simulink model "asbQuadcopters_SiFi"  (Simulink 9.1)
settings: Solver=VariableStepAuto  StartTime=0.0  StopTime=TFinal  RelTol=1e-3
values from neighbouring files (symbols this model uses):
  Controller =     [data_set.mat]
  Estimator =     [data_set.mat]
  g = 9.81    [data_set.mat]
  init =     [data_set.mat]
  rho = 1.184    [data_set.mat]
  sensorCalibrationData = [0.09 -0.06 -9.473 -0.0095 -0.0075 0.0015 101270.95 0.2]    [data_set.mat]
  Sensors =     [data_set.mat]
  States =     [data_set.mat]
  takeOffDuration = 1    [data_set.mat]
  Ts = 0.005    [data_set.mat]
  Vehicle =     [data_set.mat]
undefined symbols (not defined in the file or in its folder): DiscIntNeverNeededParam, Discrete, Earth, ft, m, s, sigbuilder_block, Time, WGS84
libraries: F_Line_block x565, simulink x39, aerolibconvert2 x4, sharedutil x3, ctrlSharedLib x3, sharedtransform x3, shared6dof x1, aerolibasang x1, aerolibtransform2 x1, aerolibnav x1, aerolibanimutils x1
(part 3 of 4)

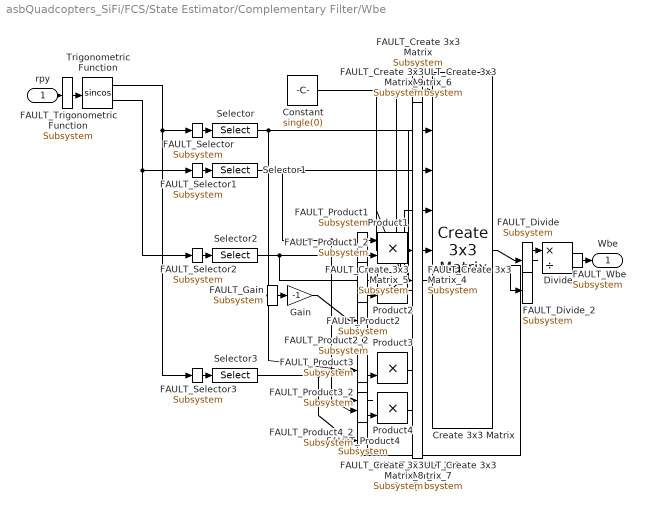
== system asbQuadcopters_SiFi/FCS/State Estimator/Complementary Filter/Wbe ==
  rpy : Inport  OutDataTypeStr=single
  Constant : Constant  Value=single(0)
  Create 3x3 Matrix : sharedutil/Create 3x3 Matrix  aMode=aMode
  FAULT_Create 3x3 Matrix : F_Line_block/Subsystem
  FAULT_Create 3x3 Matrix_{2..9} (8 alike) : F_Line_block/Subsystem
  Divide : Product  Inputs=*/
  FAULT_Divide : F_Line_block/Subsystem
  FAULT_Divide_2 : F_Line_block/Subsystem
  Gain : Gain  Gain=-1
  FAULT_Gain : F_Line_block/Subsystem
  Product{1..4} (4 alike) : Product
  FAULT_Product{1..4} (4 alike) : F_Line_block/Subsystem
  FAULT_Product1_2 : F_Line_block/Subsystem
  FAULT_Product2_2 : F_Line_block/Subsystem
  FAULT_Product3_2 : F_Line_block/Subsystem
  FAULT_Product4_2 : F_Line_block/Subsystem
  Selector : Selector  InputPortWidth=3  IndexOptions=Index vector (dialog)  Indices=[1]  OutputSizes=1
  FAULT_Selector{,1..3} (4 alike) : F_Line_block/Subsystem
  Selector1 : Selector  InputPortWidth=3  IndexOptions=Index vector (dialog)  Indices=[1]  OutputSizes=1
  Selector2 : Selector  InputPortWidth=3  IndexOptions=Index vector (dialog)  Indices=[2]  OutputSizes=1
  Selector3 : Selector  InputPortWidth=3  IndexOptions=Index vector (dialog)  Indices=[2]  OutputSizes=1
  Trigonometric Function : Trigonometry  Operator=sincos
  FAULT_Trigonometric Function : F_Line_block/Subsystem
  Wbe : Outport
  FAULT_Wbe : F_Line_block/Subsystem
  wires:
  Create 3x3 Matrix/1 -> FAULT_Divide/1
  FAULT_Divide/1 -> Divide/1
  Product3/1 -> ?
  FAULT_Create 3x3 Matrix/1 -> Create 3x3 Matrix/1
  Trigonometric Function/2 -> FAULT_Selector1/1, FAULT_Selector2/1
  FAULT_Selector1/1 -> Selector1/1
  FAULT_Selector2/1 -> Selector2/1
  Selector3/1 -> FAULT_Product4_2/1, FAULT_Product3_2/1
  FAULT_Product4_2/1 -> Product4/2
  FAULT_Product3_2/1 -> Product3/2
  Selector1/1 -> FAULT_Product4/1, Product1/1, Create 3x3 Matrix/3
  Trigonometric Function/1 -> FAULT_Selector3/1, FAULT_Selector/1
  FAULT_Selector3/1 -> Selector3/1
  FAULT_Selector/1 -> Selector/1
  Product1/1 -> FAULT_Create 3x3 Matrix_5/1
  FAULT_Create 3x3 Matrix_5/1 -> Create 3x3 Matrix/5
  Product2/1 -> ?
  FAULT_Create 3x3 Matrix_5/1 -> Create 3x3 Matrix/5
  Selector2/1 -> FAULT_Divide_2/1, Product2/1, Product1/2
  Gain/1 -> FAULT_Product2_2/1
  FAULT_Product2_2/1 -> Product2/2
  Product4/1 -> ?
  FAULT_Create 3x3 Matrix_2/1 -> Create 3x3 Matrix/2
  Constant/1 -> FAULT_Create 3x3 Matrix_4/1, FAULT_Create 3x3 Matrix/1
  FAULT_Create 3x3 Matrix_4/1 -> Create 3x3 Matrix/4
  FAULT_Create 3x3 Matrix/1 -> Create 3x3 Matrix/1
  Divide/1 -> FAULT_Wbe/1
  FAULT_Wbe/1 -> Wbe/1
  rpy/1 -> FAULT_Trigonometric Function/1
  FAULT_Trigonometric Function/1 -> Trigonometric Function/1
  Selector/1 -> FAULT_Product3/1, Gain/1, Create 3x3 Matrix/2

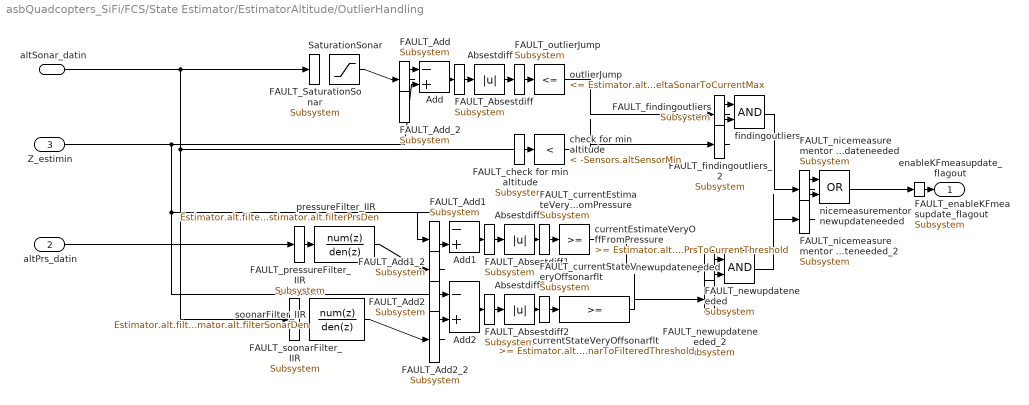
== system asbQuadcopters_SiFi/FCS/State Estimator/EstimatorAltitude/OutlierHandling ==
  altSonar_datin : Inport
  altPrs_datin : Inport  Port=2
  Z_estimin : Inport  Port=3
  Absestdiff : Abs
  FAULT_Absestdiff : F_Line_block/Subsystem
  Absestdiff1 : Abs
  FAULT_Absestdiff1 : F_Line_block/Subsystem
  Absestdiff2 : Abs
  FAULT_Absestdiff2 : F_Line_block/Subsystem
  Add : Sum  Inputs=-+
  FAULT_Add : F_Line_block/Subsystem
  FAULT_Add_2 : F_Line_block/Subsystem
  Add1 : Sum  Inputs=-+
  FAULT_Add1 : F_Line_block/Subsystem
  FAULT_Add1_2 : F_Line_block/Subsystem
  Add2 : Sum  Inputs=-+
  FAULT_Add2 : F_Line_block/Subsystem
  FAULT_Add2_2 : F_Line_block/Subsystem
  SaturationSonar : Saturate  UpperLimit=-Sensors.altSensorMin  LowerLimit=-inf
  FAULT_SaturationSonar : F_Line_block/Subsystem
  check for min altitude : simulink/Logic and Bit Operations/Compare To Constant  relop=<  const=-Sensors.altSensorMin  OutDataTypeStr=boolean
  FAULT_check for min altitude : F_Line_block/Subsystem
  currentEstimateVeryOffFromPressure : simulink/Logic and Bit Operations/Compare To Constant  relop=>=  const=Estimator.alt.deltaPrsToCurrentThreshold  OutDataTypeStr=boolean
  FAULT_currentEstimateVeryOffFromPressure : F_Line_block/Subsystem
  currentStateVeryOffsonarflt : simulink/Logic and Bit Operations/Compare To Constant  relop=>=  const=Estimator.alt.deltaSonarToFilteredThreshold  OutDataTypeStr=boolean
  FAULT_currentStateVeryOffsonarflt : F_Line_block/Subsystem
  findingoutliers : Logic  AllPortsSameDT=off  OutDataTypeStr=boolean
  FAULT_findingoutliers : F_Line_block/Subsystem
  FAULT_findingoutliers_2 : F_Line_block/Subsystem
  newupdateneeded : Logic  AllPortsSameDT=off  OutDataTypeStr=boolean
  FAULT_newupdateneeded : F_Line_block/Subsystem
  FAULT_newupdateneeded_2 : F_Line_block/Subsystem
  nicemeasurementor newupdateneeded : Logic  Operator=OR  AllPortsSameDT=off  OutDataTypeStr=boolean
  FAULT_nicemeasurementor newupdateneeded : F_Line_block/Subsystem
  FAULT_nicemeasurementor newupdateneeded_2 : F_Line_block/Subsystem
  outlierJump : simulink/Logic and Bit Operations/Compare To Constant  relop=<=  const=Estimator.alt.deltaSonarToCurrentMax  OutDataTypeStr=boolean
  FAULT_outlierJump : F_Line_block/Subsystem
  pressureFilter_IIR : DiscreteFilter  Numerator=Estimator.alt.filterPrsNum  Denominator=Estimator.alt.filterPrsDen
  FAULT_pressureFilter_IIR : F_Line_block/Subsystem
  soonarFilter_IIR : DiscreteFilter  Numerator=Estimator.alt.filterSonarNum  Denominator=Estimator.alt.filterSonarDen
  FAULT_soonarFilter_IIR : F_Line_block/Subsystem
  enableKFmeasupdate_flagout : Outport
  FAULT_enableKFmeasupdate_flagout : F_Line_block/Subsystem
  wires:
  Add1/1 -> FAULT_Absestdiff1/1
  FAULT_Absestdiff1/1 -> Absestdiff1/1
  nicemeasurementor newupdateneeded/1 -> FAULT_enableKFmeasupdate_flagout/1
  FAULT_enableKFmeasupdate_flagout/1 -> enableKFmeasupdate_flagout/1
  findingoutliers/1 -> FAULT_nicemeasurementor newupdateneeded/1
  FAULT_nicemeasurementor newupdateneeded/1 -> nicemeasurementor newupdateneeded/1
  check for min altitude/1 -> FAULT_findingoutliers_2/1
  FAULT_findingoutliers_2/1 -> findingoutliers/2
  outlierJump/1 -> FAULT_findingoutliers/1
  FAULT_findingoutliers/1 -> findingoutliers/1
  SaturationSonar/1 -> FAULT_Add/1
  FAULT_Add/1 -> Add/1
  Absestdiff/1 -> FAULT_outlierJump/1
  FAULT_outlierJump/1 -> outlierJump/1
  Add/1 -> FAULT_Absestdiff/1
  FAULT_Absestdiff/1 -> Absestdiff/1
  newupdateneeded/1 -> FAULT_nicemeasurementor newupdateneeded_2/1
  FAULT_nicemeasurementor newupdateneeded_2/1 -> nicemeasurementor newupdateneeded/2
  Absestdiff2/1 -> FAULT_currentStateVeryOffsonarflt/1
  FAULT_currentStateVeryOffsonarflt/1 -> currentStateVeryOffsonarflt/1
  altSonar_datin/1 -> FAULT_SaturationSonar/1, FAULT_soonarFilter_IIR/1, check for min altitude/1
  currentEstimateVeryOffFromPressure/1 -> FAULT_newupdateneeded/1
  FAULT_newupdateneeded/1 -> newupdateneeded/1
  Z_estimin/1 -> FAULT_Add1/1, Add2/1, Add/2
  Add2/1 -> FAULT_Absestdiff2/1
  FAULT_Absestdiff2/1 -> Absestdiff2/1
  currentStateVeryOffsonarflt/1 -> FAULT_newupdateneeded_2/1
  FAULT_newupdateneeded_2/1 -> newupdateneeded/2
  pressureFilter_IIR/1 -> FAULT_Add1_2/1
  FAULT_Add1_2/1 -> Add1/2
  altPrs_datin/1 -> FAULT_pressureFilter_IIR/1
  FAULT_pressureFilter_IIR/1 -> pressureFilter_IIR/1
  soonarFilter_IIR/1 -> FAULT_Add2_2/1
  FAULT_Add2_2/1 -> Add2/2
  Absestdiff1/1 -> FAULT_currentEstimateVeryOffFromPressure/1
  FAULT_currentEstimateVeryOffFromPressure/1 -> currentEstimateVeryOffFromPressure/1

== system asbQuadcopters_SiFi/FCS/State Estimator/EstimatorXYPosition/EstimatorVelocity ==
  opticalFlow_datin : Inport
  Z_estimin : Inport  Port=2  SampleTime=Ts
  sensorIMU_datin : Inport  Port=3
  orient_estimin : Inport  Port=4
  AccelerationHandling : Subsystem
  DataHandling : Subsystem
  Delay : Delay  DelayLength=1  InitialCondition=0
  FAULT_Delay : F_Line_block/Subsystem
  KalmanFilter_dxdy : ctrlSharedLib/Kalman Filter  TimeDomain=Discrete-Time  UseCurrentEstimator=on  ModelSource=Individual A, B, C, D matrices  ModelSourceVariable=ss(0.95,1,1,0,1)  A=eye(2)  B=Ts*eye(2)  C=eye(2)  D=0  NumberOfStates=1  NumberOfInputs=1  NumberOfOutputs=1  InitialEstimateSource=Dialog  X0=0  P0=10  UseK=off  UseGH=on  NumberOfProcessNoiseInputs=1  G=Estimator.pos.kfVelo.G  TimeInvariantG=on  H=Estimator.pos.kfVelo.H  TimeInvariantH=on  Q=Estimator.pos.kfVelo.Q  TimeInvariantQ=on  R=Estimator.pos.kfVelo.R  TimeInvariantR=on  N=Estimator.pos.kfVelo.N  TimeInvariantN=on  AddInputPort=on  AddEnablePort=on  OutputEstimatedY=off  OutputP=off  Ts=-1
      settings: SourceProductBaseCode=CT
  FAULT_KalmanFilter_dxdy : F_Line_block/Subsystem
  FAULT_KalmanFilter_dxdy_2 : F_Line_block/Subsystem
  FAULT_KalmanFilter_dxdy_3 : F_Line_block/Subsystem
  Select dxy : Selector  InputPortWidth=3  IndexOptions=Index vector (dialog)  Indices=[1 2]  OutputSizes=1
  FAULT_Select dxy : F_Line_block/Subsystem
  opticalFlowToVelocity_gain : Gain  Gain=Estimator.pos.opticalFlowToVelocityGain
  FAULT_opticalFlowToVelocity_gain : F_Line_block/Subsystem
  dxy_estimout : Outport
  FAULT_dxy_estimout : F_Line_block/Subsystem
  wires:
  Delay/1 -> DataHandling/5(dxyOF_datin)
  Z_estimin/1 -> DataHandling/1(Z_estimin), AccelerationHandling/4(Z_estimin)
  KalmanFilter_dxdy/1 -> FAULT_dxy_estimout/1, FAULT_Delay/1
  ?FAULT_Demux1/1 -> ?Demux1/1
  ?FAULT_IIRgyroz/1 -> ?IIRgyroz/1
  FAULT_dxy_estimout/1 -> dxy_estimout/1
  FAULT_Delay/1 -> Delay/1
  opticalFlowToVelocity_gain/1 -> FAULT_Select dxy/1
  FAULT_Select dxy/1 -> Select dxy/1
  opticalFlow_datin/1 -> FAULT_opticalFlowToVelocity_gain/1
  FAULT_opticalFlowToVelocity_gain/1 -> opticalFlowToVelocity_gain/1
  sensorIMU_datin/1 -> AccelerationHandling/2(sensorIMU_datin), DataHandling/3(sensorIMU_datin)
  orient_estimin/1 -> AccelerationHandling/3(orient_estimin), DataHandling/2(orient_estimin)
  Select dxy/1 -> FAULT_KalmanFilter_dxdy_2/1, AccelerationHandling/1(dxy_estimin), DataHandling/4(dxy_estimin)
  AccelerationHandling/1(acceleration_world) -> FAULT_KalmanFilter_dxdy/1
  FAULT_KalmanFilter_dxdy/1 -> KalmanFilter_dxdy/1
  DataHandling/1(enable_flag) -> FAULT_KalmanFilter_dxdy_3/1
  FAULT_KalmanFilter_dxdy_3/1 -> KalmanFilter_dxdy/3

== system asbQuadcopters_SiFi/FCS/State Estimator/EstimatorXYPosition/EstimatorXYPosition ==
  note: Switching from orientationControl to Position
      | control reset the current world position estimate
      | (happens when using no markers)
  dxy_estimin : Inport
  orient_estimin : Inport  Port=2  SampleTime=Ts
  controlModePosVSOrient_flagin : Inport  Port=3
  dz_estimin : Inport  Port=4
  posVIS_datin : Inport  Port=5
  usePosVIS_flagin : Inport  Port=6
  Delay : Delay  DelayLength=1  InitialCondition=0
  FAULT_Delay : F_Line_block/Subsystem
  KalmanFilter_posxy : ctrlSharedLib/Kalman Filter  TimeDomain=Discrete-Time  UseCurrentEstimator=on  ModelSource=Individual A, B, C, D matrices  ModelSourceVariable=ss(0.95,1,1,0,1)  A=eye(2)  B=Ts*eye(2)  C=eye(2)  D=0  NumberOfStates=1  NumberOfInputs=1  NumberOfOutputs=1  InitialEstimateSource=Dialog  X0=[.1 0]  P0=10  UseK=off  UseGH=on  NumberOfProcessNoiseInputs=1  G=Estimator.pos.kfPos.G  TimeInvariantG=on  H=Estimator.pos.kfPos.H  TimeInvariantH=on  Q=Estimator.pos.kfPos.Q  TimeInvariantQ=on  R=Estimator.pos.kfPos.R  TimeInvariantR=on  N=Estimator.pos.kfPos.N  TimeInvariantN=on  AddInputPort=on  AddEnablePort=on  OutputEstimatedY=off  OutputP=off  Ts=-1
      settings: SourceProductBaseCode=CT
  FAULT_KalmanFilter_posxy : F_Line_block/Subsystem
  FAULT_KalmanFilter_posxy_2 : F_Line_block/Subsystem
  FAULT_KalmanFilter_posxy_3 : F_Line_block/Subsystem
  Math Function : Math  Operator=transpose  SaturateOnIntegerOverflow=on
  FAULT_Math Function : F_Line_block/Subsystem
  Mux2 : Mux  Inputs=2
  FAULT_Mux2 : F_Line_block/Subsystem
  FAULT_Mux2_2 : F_Line_block/Subsystem
  OutlierHandling : Subsystem
  Product : Product  Multiplication=Matrix(*)
  FAULT_Product : F_Line_block/Subsystem
  FAULT_Product_2 : F_Line_block/Subsystem
  Rotation Angles to Direction Cosine Matrix : sharedtransform/Rotation Angles to Direction Cosine Matrix  rotationOrder=ZYX  aMode=aMode
      settings: SourceProductBaseCode=AE
  FAULT_Rotation Angles to Direction Cosine Matrix : F_Line_block/Subsystem
  SelectXY : Selector  InputPortWidth=4  IndexOptions=Index vector (dialog)  Indices=[1 2]  OutputSizes=1
  FAULT_SelectXY : F_Line_block/Subsystem
  SelectdXY : Selector  InputPortWidth=3  IndexOptions=Index vector (dialog)  Indices=[1 2]  OutputSizes=1
  FAULT_SelectdXY : F_Line_block/Subsystem
  SimplyIntegrateVelocity : DiscreteIntegrator  ExternalReset=rising  SampleTime=Ts  ICPrevOutput=DiscIntNeverNeededParam  ICPrevScaledInput=DiscIntNeverNeededParam
  FAULT_SimplyIntegrateVelocity : F_Line_block/Subsystem
  FAULT_SimplyIntegrateVelocity_2 : F_Line_block/Subsystem
  UseIPPosSwitch : Switch  Criteria=u2 > Threshold
  XY_estimout : Outport
  FAULT_XY_estimout : F_Line_block/Subsystem
  wires:
  Delay/1 -> OutlierHandling/3(pos_estim)
  usePosVIS_flagin/1 -> UseIPPosSwitch/2
  UseIPPosSwitch/1 -> FAULT_XY_estimout/1
  FAULT_XY_estimout/1 -> XY_estimout/1
  controlModePosVSOrient_flagin/1 -> FAULT_SimplyIntegrateVelocity_2/1
  FAULT_SimplyIntegrateVelocity_2/1 -> SimplyIntegrateVelocity/2
  KalmanFilter_posxy/1 -> FAULT_Delay/1, UseIPPosSwitch/1
  FAULT_Delay/1 -> Delay/1
  FAULT_SelectXY/1 -> SelectXY/1
  posVIS_datin/1 -> OutlierHandling/2(posVIS_datin), FAULT_SelectXY/1
  FAULT_Delay/1 -> Delay/1
  FAULT_SelectXY/1 -> SelectXY/1
  Product/1 -> FAULT_SelectdXY/1
  FAULT_SelectdXY/1 -> SelectdXY/1
  Mux2/1 -> FAULT_Product_2/1
  FAULT_Product_2/1 -> Product/2
  dz_estimin/1 -> FAULT_Mux2_2/1
  FAULT_Mux2_2/1 -> Mux2/2
  SimplyIntegrateVelocity/1 -> UseIPPosSwitch/3
  dxy_estimin/1 -> FAULT_Mux2/1
  FAULT_Mux2/1 -> Mux2/1
  orient_estimin/1 -> FAULT_Rotation Angles to Direction Cosine Matrix/1, OutlierHandling/1(orient_estimin)
  FAULT_Rotation Angles to Direction Cosine Matrix/1 -> Rotation Angles to Direction Cosine Matrix/1
  FAULT_SelectXY/1 -> SelectXY/1
  Rotation Angles to Direction Cosine Matrix/1 -> FAULT_Math Function/1
  FAULT_Math Function/1 -> Math Function/1
  SelectXY/1 -> FAULT_KalmanFilter_posxy_2/1
  FAULT_KalmanFilter_posxy_2/1 -> KalmanFilter_posxy/2
  OutlierHandling/1(enable_flag) -> FAULT_KalmanFilter_posxy_3/1
  FAULT_KalmanFilter_posxy_3/1 -> KalmanFilter_posxy/3
  SelectdXY/1 -> FAULT_SimplyIntegrateVelocity/1, FAULT_KalmanFilter_posxy/1
  FAULT_SimplyIntegrateVelocity/1 -> SimplyIntegrateVelocity/1
  FAULT_KalmanFilter_posxy/1 -> KalmanFilter_posxy/1
  Math Function/1 -> FAULT_Product/1
  FAULT_Product/1 -> Product/1

== system asbQuadcopters_SiFi/Sensor/Sensor System/IMU_Pressure/HAL_acquisition_creator ==
  sensors : Inport
  Bus Creator4 : BusCreator  Inputs=21  OutDataTypeStr=Bus: HAL_acquisition_t  NonVirtualBus=on
      settings: InheritFromInputs=off
  Demux3 : Demux  Outputs=8
  HAL_acc_SI_creator : Subsystem
  HAL_fifo_fsync : Constant  Value=zeros(5,1)  OutDataTypeStr=uint8
  HAL_fifo_gyro_SI_t_creator : Subsystem
  HAL_fifo_gyro_SI_t_creator1 : Subsystem
  HAL_fifo_gyro_SI_t_creator2 : Subsystem
  HAL_fifo_gyro_SI_t_creator3 : Subsystem
  HAL_gyro_SI_creator : Subsystem
  HAL_magn_mG_t_creator1 : Subsystem
  HAL_pressure_SI_creator : Subsystem
  HAL_ultrasound_SI_creator : Subsystem
  HAL_vbat_SI_creator : Subsystem
  number_HAL_read_call : Constant  Value=0  OutDataTypeStr=int32
  number_HAL_read_call1 : Constant  Value=0  OutDataTypeStr=uint32
  number_HAL_read_call2 : Constant  Value=0  OutDataTypeStr=uint16
  number_HAL_read_call3 : Constant  Value=0  OutDataTypeStr=uint8
  number_HAL_read_call4 : Constant  Value=0  OutDataTypeStr=uint8
  number_HAL_read_call5 : Constant  Value=0  OutDataTypeStr=uint16
  number_HAL_read_call6 : Constant  Value=0  OutDataTypeStr=uint32
  number_HAL_read_call7 : Constant  Value=0  OutDataTypeStr=single
  number_HAL_read_call8 : Constant  Value=0  OutDataTypeStr=int32
  padding : Constant  Value=zeros(1,196)  OutDataTypeStr=uint8
  HAL_acquisition_t : Outport  OutDataTypeStr=Bus: HAL_acquisition_t
  wires:
  Demux3/4 -> HAL_gyro_SI_creator/1(x)  "x"
  HAL_gyro_SI_creator/1(HAL_gyro_SI) -> Bus Creator4/7  "HAL_gyro_SI"
  Demux3/7 -> HAL_ultrasound_SI_creator/1(altitude)  "altitude"
  HAL_fifo_gyro_SI_t_creator2/1(HAL_fifo_gyro_SI_TempCorr) -> Bus Creator4/12  "HAL_fifo_gyro_SI"
  HAL_magn_mG_t_creator1/1(HAL_magn_mG) -> Bus Creator4/17  "HAL_magn_mG"
  HAL_vbat_SI_creator/1(HAL_vbat_SI) -> Bus Creator4/21  "HAL_vbat_SI"
  sensors/1 -> Demux3/1
  number_HAL_read_call4/1 -> Bus Creator4/5  "count_user"
  Demux3/5 -> HAL_gyro_SI_creator/2(y)  "y"
  number_HAL_read_call8/1 -> Bus Creator4/16  "HAL_fifo_size"
  HAL_fifo_gyro_SI_t_creator1/1(HAL_fifo_acce_SI_TempCorr) -> Bus Creator4/11  "HAL_fifo_acce_SI_TempCorr"
  Demux3/6 -> HAL_gyro_SI_creator/3(z)  "z"
  Demux3/8 -> HAL_pressure_SI_creator/1(pressure)  "pressure"
  number_HAL_read_call/1 -> Bus Creator4/1  "number_HAL_read_call"
  number_HAL_read_call6/1 -> Bus Creator4/9  "fifo_timestamp"
  number_HAL_read_call3/1 -> Bus Creator4/4  "used"
  number_HAL_read_call5/1 -> Bus Creator4/8  "HAL_fifo_count"
  Demux3/2 -> HAL_acc_SI_creator/2(y)  "y"
  number_HAL_read_call2/1 -> Bus Creator4/3  "status"
  Demux3/1 -> HAL_acc_SI_creator/1(x)  "x"
  padding/1 -> Bus Creator4/20  "padding"
  HAL_fifo_fsync/1 -> Bus Creator4/15  "HAL_fifo_fsync"
  number_HAL_read_call7/1 -> Bus Creator4/14  "HAL_ref_IMU_temp"
  number_HAL_read_call1/1 -> Bus Creator4/2  "timestamp"
  HAL_fifo_gyro_SI_t_creator3/1(HAL_fifo_acce_SI_TempCorr) -> Bus Creator4/13  "HAL_fifo_acce_SI"
  HAL_acc_SI_creator/1(HAL_acc_SI) -> Bus Creator4/6  "HAL_acc_SI"
  HAL_fifo_gyro_SI_t_creator/1(HAL_fifo_gyro_SI_TempCorr) -> Bus Creator4/10  "HAL_fifo_gyro_SI_TempCorr"
  Demux3/3 -> HAL_acc_SI_creator/3(z)  "z"
  HAL_pressure_SI_creator/1(HAL_pressure_SI) -> Bus Creator4/18  "HAL_pressure_SI"
  Bus Creator4/1 -> HAL_acquisition_t/1  "HAL_acquisition_t"
  HAL_ultrasound_SI_creator/1(HAL_ultrasound_SI) -> Bus Creator4/19  "HAL_ultrasound_SI"

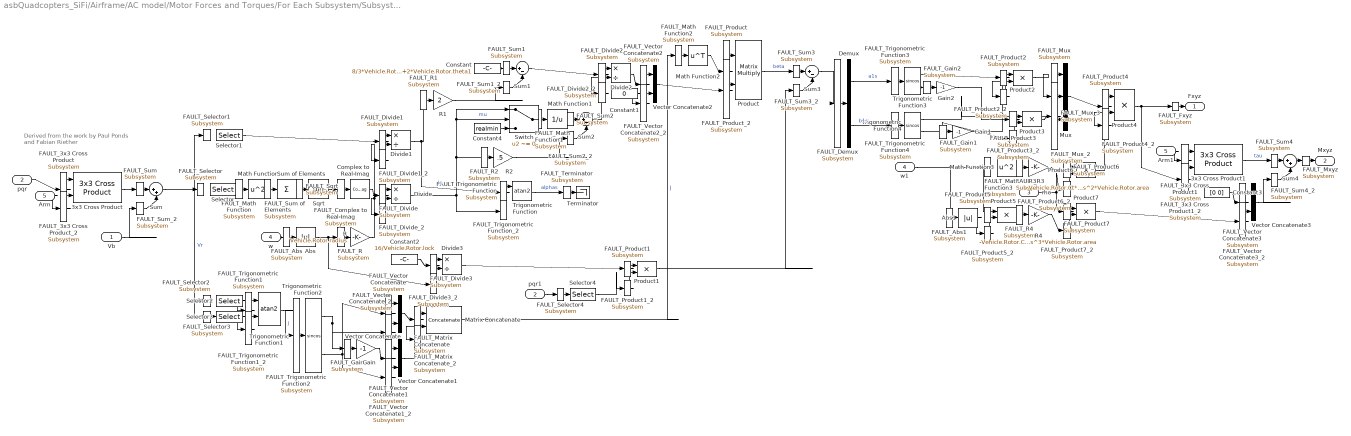
== system asbQuadcopters_SiFi/Airframe/AC model/Motor Forces and Torques/For Each Subsystem/Subsystem ==
  note: Derived from the work by Paul Ponds
      | and Fabian Riether
  Vb : Inport  PortDimensions=3
  pqr : Inport  Port=2  PortDimensions=3
  rho : Inport  Port=3  PortDimensions=1
  w : Inport  Port=4  PortDimensions=[1 1]
  Arm : Inport  Port=5  PortDimensions=[3 1]
  3x3 Cross Product : sharedutil/3x3 Cross Product  aMode=aMode
      settings: SourceProductBaseCode=AE
  FAULT_3x3 Cross Product : F_Line_block/Subsystem
  FAULT_3x3 Cross Product_2 : F_Line_block/Subsystem
  3x3 Cross Product1 : sharedutil/3x3 Cross Product  aMode=aMode
      settings: SourceProductBaseCode=AE
  FAULT_3x3 Cross Product1 : F_Line_block/Subsystem
  FAULT_3x3 Cross Product1_2 : F_Line_block/Subsystem
  Abs : Abs
  FAULT_Abs : F_Line_block/Subsystem
  Abs1 : Abs
  FAULT_Abs1 : F_Line_block/Subsystem
  Arm1 : InportShadow  Port=5  PortDimensions=[3 1]
  Complex to Real-Imag : ComplexToRealImag  Output=Real
  FAULT_Complex to Real-Imag : F_Line_block/Subsystem
  Constant : Constant  Value=8/3*Vehicle.Rotor.theta0+2*Vehicle.Rotor.theta1
  Constant1 : Constant  Value=0
  Constant2 : Constant  Value=16/Vehicle.Rotor.lock
  Constant3 : Constant  Value=[0 0]
  Constant4 : Constant  Value=realmin
  Demux : Demux  Outputs=2
  FAULT_Demux : F_Line_block/Subsystem
  Divide{,1..3} (4 alike) : Product  Inputs=*/
  FAULT_Divide{,1..3} (4 alike) : F_Line_block/Subsystem
  FAULT_Divide_2 : F_Line_block/Subsystem
  FAULT_Divide1_2 : F_Line_block/Subsystem
  FAULT_Divide2_2 : F_Line_block/Subsystem
  FAULT_Divide3_2 : F_Line_block/Subsystem
  Gain : Gain  Gain=-1
  FAULT_Gain : F_Line_block/Subsystem
  Gain1 : Gain  Gain=-1
  FAULT_Gain1 : F_Line_block/Subsystem
  Gain2 : Gain  Gain=-1
  FAULT_Gain2 : F_Line_block/Subsystem
  Math Function : Math  Operator=square  SaturateOnIntegerOverflow=on
  FAULT_Math Function{,1..3} (4 alike) : F_Line_block/Subsystem
  Math Function1 : Math  Operator=reciprocal  SaturateOnIntegerOverflow=on
  Math Function2 : Math  Operator=transpose  SaturateOnIntegerOverflow=on
  Math Function3 : Math  Operator=square  SaturateOnIntegerOverflow=on
  Matrix Concatenate : Concatenate  Mode=Multidimensional array  ConcatenateDimension=2
  FAULT_Matrix Concatenate : F_Line_block/Subsystem
  FAULT_Matrix Concatenate_2 : F_Line_block/Subsystem
  Mux : Mux  Inputs=3
  FAULT_Mux : F_Line_block/Subsystem
  FAULT_Mux_2 : F_Line_block/Subsystem
  FAULT_Mux_3 : F_Line_block/Subsystem
  Product : Product  Multiplication=Matrix(*)
  FAULT_Product{,1..7} (8 alike) : F_Line_block/Subsystem
  FAULT_Product_2 : F_Line_block/Subsystem
  Product{1..7} (7 alike) : Product
  FAULT_Product1_2 : F_Line_block/Subsystem
  FAULT_Product2_2 : F_Line_block/Subsystem
  FAULT_Product3_2 : F_Line_block/Subsystem
  FAULT_Product4_2 : F_Line_block/Subsystem
  FAULT_Product5_2 : F_Line_block/Subsystem
  FAULT_Product6_2 : F_Line_block/Subsystem
  FAULT_Product7_2 : F_Line_block/Subsystem
  R : Gain  Gain=Vehicle.Rotor.radius
  FAULT_R{,1..4} (5 alike) : F_Line_block/Subsystem
  R1 : Gain  Gain=2
  R2 : Gain  Gain=.5
  R3 : Gain  Gain=Vehicle.Rotor.Ct*Vehicle.Rotor.radius^2*Vehicle.Rotor.area
  R4 : Gain  Gain=-Vehicle.Rotor.Cq*Vehicle.Rotor.radius^3*Vehicle.Rotor.area
  Selector : Selector  InputPortWidth=3  IndexOptions=Index vector (dialog)  Indices=[1 2]  OutputSizes=1
  FAULT_Selector{,1..4} (5 alike) : F_Line_block/Subsystem
  Selector1 : Selector  InputPortWidth=3  IndexOptions=Index vector (dialog)  Indices=[3]  OutputSizes=1
  Selector2 : Selector  InputPortWidth=3  IndexOptions=Index vector (dialog)  Indices=[2]  OutputSizes=1
  Selector3 : Selector  InputPortWidth=3  IndexOptions=Index vector (dialog)  Indices=[1]  OutputSizes=1
  Selector4 : Selector  InputPortWidth=3  IndexOptions=Index vector (dialog)  Indices=[2 1]  OutputSizes=1
  Sqrt : Sqrt  OutputSignalType=complex  SaturateOnIntegerOverflow=on
  FAULT_Sqrt : F_Line_block/Subsystem
  Sum : Sum  Inputs=|++
  FAULT_Sum{,1..4} (5 alike) : F_Line_block/Subsystem
  FAULT_Sum_2 : F_Line_block/Subsystem
  Sum of Elements : Sum  Inputs=+
  FAULT_Sum of Elements : F_Line_block/Subsystem
  Sum1 : Sum  Inputs=|+-
  FAULT_Sum1_2 : F_Line_block/Subsystem
  Sum2 : Sum  Inputs=|+-
  FAULT_Sum2_2 : F_Line_block/Subsystem
  Sum3 : Sum  Inputs=|+-
  FAULT_Sum3_2 : F_Line_block/Subsystem
  Sum4 : Sum  Inputs=|++
  FAULT_Sum4_2 : F_Line_block/Subsystem
  Switch : Switch  Criteria=u2 ~= 0
  Terminator : Terminator
  FAULT_Terminator : F_Line_block/Subsystem
  Trigonometric Function : Trigonometry  Operator=atan2
  FAULT_Trigonometric Function{,1..4} (5 alike) : F_Line_block/Subsystem
  FAULT_Trigonometric Function_2 : F_Line_block/Subsystem
  Trigonometric Function1 : Trigonometry  Operator=atan2
  FAULT_Trigonometric Function1_2 : F_Line_block/Subsystem
  Trigonometric Function2 : Trigonometry  Operator=sincos
  Trigonometric Function3 : Trigonometry  Operator=sincos
  Trigonometric Function4 : Trigonometry  Operator=sincos
  Vector Concatenate{,1..3} (4 alike) : Concatenate
  FAULT_Vector Concatenate{,1..3} (4 alike) : F_Line_block/Subsystem
  FAULT_Vector Concatenate_2 : F_Line_block/Subsystem
  FAULT_Vector Concatenate1_2 : F_Line_block/Subsystem
  FAULT_Vector Concatenate2_2 : F_Line_block/Subsystem
  FAULT_Vector Concatenate3_2 : F_Line_block/Subsystem
  pqr1 : InportShadow  Port=2  PortDimensions=3
  w1 : InportShadow  Port=4  PortDimensions=[1 1]
  Fxyz : Outport  PortDimensions=[3 1]
  FAULT_Fxyz : F_Line_block/Subsystem
  Mxyz : Outport  Port=2  PortDimensions=[3 1]
  FAULT_Mxyz : F_Line_block/Subsystem
  wires:
  Product4/1 -> FAULT_Fxyz/1, FAULT_3x3 Cross Product1_2/1
  FAULT_Fxyz/1 -> Fxyz/1
  FAULT_3x3 Cross Product1_2/1 -> 3x3 Cross Product1/2
  3x3 Cross Product/1 -> FAULT_Sum/1
  FAULT_Sum/1 -> Sum/1
  Matrix Concatenate/1 -> FAULT_Math Function2/1  "J"
  FAULT_Math Function2/1 -> Math Function2/1
  Divide1/1 -> FAULT_Trigonometric Function/1, FAULT_R1/1  "lc"
  FAULT_Trigonometric Function/1 -> Trigonometric Function/1
  FAULT_R1/1 -> R1/1
  w/1 -> FAULT_Abs/1
  FAULT_Abs/1 -> Abs/1
  Product7/1 -> FAULT_Vector Concatenate3_2/1
  FAULT_Vector Concatenate3_2/1 -> Vector Concatenate3/2
  Sum/1 -> FAULT_Selector/1, FAULT_Selector1/1, FAULT_Selector2/1, Selector3/1  "Vr"
  Abs/1 -> FAULT_R/1, FAULT_Divide3_2/1
  FAULT_R/1 -> R/1
  FAULT_Divide3_2/1 -> Divide3/2
  Math Function1/1 -> FAULT_Sum2/1
  FAULT_Sum2/1 -> Sum2/1
  R2/1 -> FAULT_Sum2_2/1
  FAULT_Sum2_2/1 -> Sum2/2
  Selector1/1 -> FAULT_Divide1/1
  FAULT_Divide1/1 -> Divide1/1
  Selector/1 -> FAULT_Math Function/1
  FAULT_Math Function/1 -> Math Function/1
  R/1 -> FAULT_Divide_2/1, FAULT_Divide1_2/1
  FAULT_Divide_2/1 -> Divide/2
  FAULT_Divide1_2/1 -> Divide1/2
  Arm/1 -> FAULT_3x3 Cross Product_2/1
  FAULT_3x3 Cross Product_2/1 -> 3x3 Cross Product/2
  pqr/1 -> FAULT_3x3 Cross Product/1
  FAULT_3x3 Cross Product/1 -> 3x3 Cross Product/1
  Product2/1 -> FAULT_Mux/1
  FAULT_Mux/1 -> Mux/1
  Trigonometric Function3/2 -> FAULT_Gain2/1
  FAULT_Gain2/1 -> Gain2/1
  Vector Concatenate/1 -> FAULT_Matrix Concatenate/1
  FAULT_Matrix Concatenate/1 -> Matrix Concatenate/1
  Gain1/1 -> FAULT_Product2_2/1
  FAULT_Product2_2/1 -> Product2/2
  Vector Concatenate1/1 -> FAULT_Matrix Concatenate_2/1
  FAULT_Matrix Concatenate_2/1 -> Matrix Concatenate/2
  Sum2/1 -> FAULT_Divide2_2/1
  FAULT_Divide2_2/1 -> Divide2/2
  Trigonometric Function2/1 -> FAULT_Gain/1, FAULT_Vector Concatenate_2/1
  FAULT_Gain/1 -> Gain/1
  FAULT_Vector Concatenate_2/1 -> Vector Concatenate/2
  Sum1/1 -> FAULT_Divide2/1
  FAULT_Divide2/1 -> Divide2/1
  Trigonometric Function3/1 -> FAULT_Product2/1
  FAULT_Product2/1 -> Product2/1
  Constant1/1 -> FAULT_Vector Concatenate2_2/1
  FAULT_Vector Concatenate2_2/1 -> Vector Concatenate2/2
  3x3 Cross Product1/1 -> FAULT_Sum4/1  "tau"
  FAULT_Sum4/1 -> Sum4/1
  Math Function3/1 -> FAULT_R3/1
  FAULT_R3/1 -> R3/1
  Demux/2 -> FAULT_Trigonometric Function4/1  "b1s"
  FAULT_Trigonometric Function4/1 -> Trigonometric Function4/1
  Trigonometric Function2/2 -> FAULT_Vector Concatenate/1, FAULT_Vector Concatenate1_2/1
  FAULT_Vector Concatenate/1 -> Vector Concatenate/1
  FAULT_Vector Concatenate1_2/1 -> Vector Concatenate1/2
  pqr1/1 -> FAULT_Selector4/1
  FAULT_Selector4/1 -> Selector4/1
  Gain/1 -> FAULT_Vector Concatenate1/1
  FAULT_Vector Concatenate1/1 -> Vector Concatenate1/1
  Selector3/1 -> FAULT_Trigonometric Function1_2/1
  FAULT_Trigonometric Function1_2/1 -> Trigonometric Function1/2
  Selector2/1 -> FAULT_Trigonometric Function1/1
  FAULT_Trigonometric Function1/1 -> Trigonometric Function1/1
  Product3/1 -> FAULT_Mux_3/1
  FAULT_Mux_3/1 -> Mux/3
  R1/1 -> FAULT_Sum1_2/1
  FAULT_Sum1_2/1 -> Sum1/2
  Trigonometric Function1/1 -> FAULT_Trigonometric Function2/1  "j"
  FAULT_Trigonometric Function2/1 -> Trigonometric Function2/1
  Constant2/1 -> FAULT_Divide3/1
  FAULT_Divide3/1 -> Divide3/1
  Sum of Elements/1 -> FAULT_Sqrt/1
  FAULT_Sqrt/1 -> Sqrt/1
  Trigonometric Function/1 -> FAULT_Terminator/1  "alphas"
  FAULT_Terminator/1 -> Terminator/1
  Constant/1 -> FAULT_Sum1/1
  FAULT_Sum1/1 -> Sum1/1
  Divide3/1 -> FAULT_Product1/1
  FAULT_Product1/1 -> Product1/1
  Selector4/1 -> FAULT_Product1_2/1
  FAULT_Product1_2/1 -> Product1/2
  Abs1/1 -> FAULT_Product5_2/1
  FAULT_Product5_2/1 -> Product5/2
  Product/1 -> FAULT_Sum3/1  "beta"
  FAULT_Sum3/1 -> Sum3/1
  Vector Concatenate2/1 -> FAULT_Product_2/1
  FAULT_Product_2/1 -> Product/2
  Divide2/1 -> FAULT_Vector Concatenate2/1
  FAULT_Vector Concatenate2/1 -> Vector Concatenate2/1
  Product6/1 -> FAULT_Product4_2/1
  FAULT_Product4_2/1 -> Product4/2
  Trigonometric Function4/1 -> FAULT_Mux_2/1
  FAULT_Mux_2/1 -> Mux/2
  Mux/1 -> FAULT_Product4/1
  FAULT_Product4/1 -> Product4/1
  Vb/1 -> FAULT_Sum_2/1
  FAULT_Sum_2/1 -> Sum/2
  Vector Concatenate3/1 -> FAULT_Sum4_2/1
  FAULT_Sum4_2/1 -> Sum4/2
  R4/1 -> FAULT_Product7_2/1
  FAULT_Product7_2/1 -> Product7/2
  Divide/1 -> FAULT_Trigonometric Function_2/1, Switch/1, Switch/2, R2/1  "mu"
  Complex to Real-Imag/1 -> FAULT_Divide/1
  FAULT_Divide/1 -> Divide/1
  Math Function2/1 -> FAULT_Product/1
  FAULT_Product/1 -> Product/1
  Sum4/1 -> FAULT_Mxyz/1
  FAULT_Mxyz/1 -> Mxyz/1
  Math Function/1 -> FAULT_Sum of Elements/1
  FAULT_Sum of Elements/1 -> Sum of Elements/1
  Demux/1 -> FAULT_Trigonometric Function3/1  "a1s"
  FAULT_Trigonometric Function3/1 -> Trigonometric Function3/1
  Gain2/1 -> FAULT_Product3/1
  FAULT_Product3/1 -> Product3/1
  Sum3/1 -> FAULT_Demux/1
  FAULT_Demux/1 -> Demux/1
  Switch/1 -> FAULT_Math Function1/1
  FAULT_Math Function1/1 -> Math Function1/1
  Product5/1 -> FAULT_R4/1
  FAULT_R4/1 -> R4/1
  Product1/1 -> FAULT_Sum3_2/1
  FAULT_Sum3_2/1 -> Sum3/2
  Constant3/1 -> FAULT_Vector Concatenate3/1
  FAULT_Vector Concatenate3/1 -> Vector Concatenate3/1
  Trigonometric Function4/2 -> FAULT_Gain1/1, FAULT_Product3_2/1
  FAULT_Gain1/1 -> Gain1/1
  FAULT_Product3_2/1 -> Product3/2
  w1/1 -> FAULT_Math Function3/1, Product5/1, Abs1/1
  rho/1 -> FAULT_Product7/1, FAULT_Product6_2/1
  FAULT_Product7/1 -> Product7/1
  FAULT_Product6_2/1 -> Product6/2
  Constant4/1 -> Switch/3
  Arm1/1 -> FAULT_3x3 Cross Product1/1
  FAULT_3x3 Cross Product1/1 -> 3x3 Cross Product1/1
  Sqrt/1 -> FAULT_Complex to Real-Imag/1
  FAULT_Complex to Real-Imag/1 -> Complex to Real-Imag/1
  R3/1 -> FAULT_Product6/1
  FAULT_Product6/1 -> Product6/1

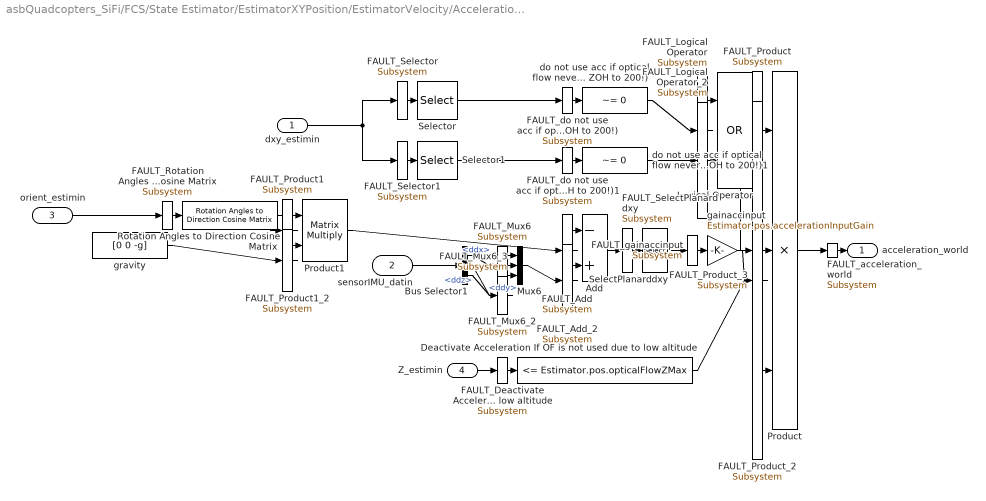
== system asbQuadcopters_SiFi/FCS/State Estimator/EstimatorXYPosition/EstimatorVelocity/AccelerationHandling ==
  dxy_estimin : Inport
  sensorIMU_datin : Inport  Port=2
  orient_estimin : Inport  Port=3
  Z_estimin : Inport  Port=4
  Add : Sum  Inputs=-+
  FAULT_Add : F_Line_block/Subsystem
  FAULT_Add_2 : F_Line_block/Subsystem
  Bus Selector1 : BusSelector  OutputSignals=ddx,ddy,ddz
  Deactivate Acceleration If OF is not used due to low altitude : simulink/Logic and Bit Operations/Compare To Constant  relop=<=  const=Estimator.pos.opticalFlowZMax  OutDataTypeStr=boolean
  FAULT_Deactivate Acceleration If OF is not used due to low altitude : F_Line_block/Subsystem
  Logical Operator : Logic  Operator=OR  AllPortsSameDT=off  OutDataTypeStr=boolean
  FAULT_Logical Operator : F_Line_block/Subsystem
  FAULT_Logical Operator_2 : F_Line_block/Subsystem
  Mux6 : Mux  Inputs=3
  FAULT_Mux6 : F_Line_block/Subsystem
  FAULT_Mux6_2 : F_Line_block/Subsystem
  FAULT_Mux6_3 : F_Line_block/Subsystem
  Product : Product  Inputs=3
  FAULT_Product : F_Line_block/Subsystem
  FAULT_Product_2 : F_Line_block/Subsystem
  FAULT_Product_3 : F_Line_block/Subsystem
  Product1 : Product  Multiplication=Matrix(*)
  FAULT_Product1 : F_Line_block/Subsystem
  FAULT_Product1_2 : F_Line_block/Subsystem
  Rotation Angles to Direction Cosine Matrix : sharedtransform/Rotation Angles to Direction Cosine Matrix  rotationOrder=ZYX  aMode=aMode
      settings: SourceProductBaseCode=AE
  FAULT_Rotation Angles to Direction Cosine Matrix : F_Line_block/Subsystem
  SelectPlanarddxy : Selector  InputPortWidth=3  IndexOptions=Index vector (dialog)  Indices=[1 2]  OutputSizes=1
  FAULT_SelectPlanarddxy : F_Line_block/Subsystem
  Selector : Selector  InputPortWidth=2  IndexOptions=Index vector (dialog)  Indices=1  OutputSizes=1
  FAULT_Selector : F_Line_block/Subsystem
  Selector1 : Selector  InputPortWidth=2  IndexOptions=Index vector (dialog)  Indices=2  OutputSizes=1
  FAULT_Selector1 : F_Line_block/Subsystem
  do not use acc if optical flow never available (Note OF@60Hz but ZOH to 200!) : simulink/Logic and Bit Operations/Compare To Constant  relop=~=  const=0  OutDataTypeStr=boolean
  FAULT_do not use acc if optical flow never available (Note OF@60Hz but ZOH to 200!) : F_Line_block/Subsystem
  do not use acc if optical flow never available (Note OF@60Hz but ZOH to 200!)1 : simulink/Logic and Bit Operations/Compare To Constant  relop=~=  const=0  OutDataTypeStr=boolean
  FAULT_do not use acc if optical flow never available (Note OF@60Hz but ZOH to 200!)1 : F_Line_block/Subsystem
  gainaccinput : Gain  Gain=Estimator.pos.accelerationInputGain  OutDataTypeStr=single
  FAULT_gainaccinput : F_Line_block/Subsystem
  gravity : Constant  Value=[0 0 -g]
  acceleration_world : Outport  OutDataTypeStr=single
  FAULT_acceleration_world : F_Line_block/Subsystem
  wires:
  do not use acc if optical flow never available (Note OF@60Hz but ZOH to 200!)1/1 -> FAULT_Logical Operator_2/1
  FAULT_Logical Operator_2/1 -> Logical Operator/2
  do not use acc if optical flow never available (Note OF@60Hz but ZOH to 200!)/1 -> FAULT_Logical Operator/1
  FAULT_Logical Operator/1 -> Logical Operator/1
  Logical Operator/1 -> FAULT_Product/1
  FAULT_Product/1 -> Product/1
  Selector1/1 -> FAULT_do not use acc if optical flow never available (Note OF@60Hz but ZOH to 200!)1/1
  FAULT_do not use acc if optical flow never available (Note OF@60Hz but ZOH to 200!)1/1 -> do not use acc if optical flow never available (Note OF@60Hz but ZOH to 200!)1/1
  Selector/1 -> FAULT_do not use acc if optical flow never available (Note OF@60Hz but ZOH to 200!)/1
  FAULT_do not use acc if optical flow never available (Note OF@60Hz but ZOH to 200!)/1 -> do not use acc if optical flow never available (Note OF@60Hz but ZOH to 200!)/1
  dxy_estimin/1 -> FAULT_Selector1/1, FAULT_Selector/1
  FAULT_Selector1/1 -> Selector1/1
  FAULT_Selector/1 -> Selector/1
  Product/1 -> FAULT_acceleration_world/1
  FAULT_acceleration_world/1 -> acceleration_world/1
  Deactivate Acceleration If OF is not used due to low altitude/1 -> FAULT_Product_3/1
  FAULT_Product_3/1 -> Product/3
  Z_estimin/1 -> FAULT_Deactivate Acceleration If OF is not used due to low altitude/1
  FAULT_Deactivate Acceleration If OF is not used due to low altitude/1 -> Deactivate Acceleration If OF is not used due to low altitude/1
  Add/1 -> FAULT_SelectPlanarddxy/1
  FAULT_SelectPlanarddxy/1 -> SelectPlanarddxy/1
  Product1/1 -> FAULT_Add/1
  FAULT_Add/1 -> Add/1
  gravity/1 -> FAULT_Product1_2/1
  FAULT_Product1_2/1 -> Product1/2
  gainaccinput/1 -> FAULT_Product_2/1
  FAULT_Product_2/1 -> Product/2
  SelectPlanarddxy/1 -> FAULT_gainaccinput/1
  FAULT_gainaccinput/1 -> gainaccinput/1
  Bus Selector1/3 -> FAULT_Mux6_3/1  "<ddz>"
  FAULT_Mux6_3/1 -> Mux6/3
  Bus Selector1/1 -> FAULT_Mux6/1  "<ddx>"
  FAULT_Mux6/1 -> Mux6/1
  sensorIMU_datin/1 -> Bus Selector1/1
  Mux6/1 -> FAULT_Add_2/1
  FAULT_Add_2/1 -> Add/2
  Bus Selector1/2 -> FAULT_Mux6_2/1  "<ddy>"
  FAULT_Mux6_2/1 -> Mux6/2
  orient_estimin/1 -> FAULT_Rotation Angles to Direction Cosine Matrix/1
  FAULT_Rotation Angles to Direction Cosine Matrix/1 -> Rotation Angles to Direction Cosine Matrix/1
  Rotation Angles to Direction Cosine Matrix/1 -> FAULT_Product1/1
  FAULT_Product1/1 -> Product1/1

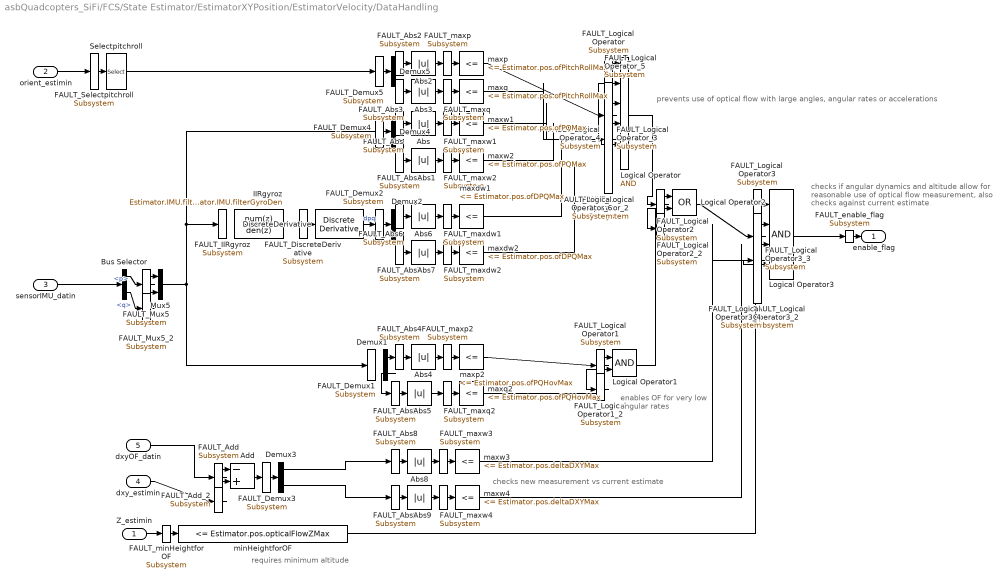
== system asbQuadcopters_SiFi/FCS/State Estimator/EstimatorXYPosition/EstimatorVelocity/DataHandling ==
  note: prevents use of optical flow with large angles, angular rates or accelerations
  note: enables OF for very
      | low angular rates
  note: checks if angular dynamics and altitude allow for
      | reasonable use of optical flow measurement,
      | also checks against current estimate
  note: checks new measurement vs current estimate
  note: requires minimum altitude
  Z_estimin : Inport
  orient_estimin : Inport  Port=2
  sensorIMU_datin : Inport  Port=3
  dxy_estimin : Inport  Port=4
  dxyOF_datin : Inport  Port=5
  Abs{,1..9} (10 alike) : Abs
  FAULT_Abs{,1..9} (10 alike) : F_Line_block/Subsystem
  Add : Sum  Inputs=-+
  FAULT_Add : F_Line_block/Subsystem
  FAULT_Add_2 : F_Line_block/Subsystem
  Bus Selector : BusSelector  OutputSignals=p,q
  Demux{1..5} (5 alike) : Demux  Outputs=2
  FAULT_Demux{1..5} (5 alike) : F_Line_block/Subsystem
  DiscreteDerivative : simulink/Discrete/Discrete Derivative  gainval=1.0  ICPrevScaledInput=0.0  InputProcessing=Inherited  OutMin=[]  OutMax=[]  OutDataType=fixdt(1, 16)  OutScaling=2^-10  DoSatur=off
  FAULT_DiscreteDerivative : F_Line_block/Subsystem
  IIRgyroz : DiscreteFilter  Numerator=Estimator.IMU.filterGyroNum  Denominator=Estimator.IMU.filterGyroDen
  FAULT_IIRgyroz : F_Line_block/Subsystem
  Logical Operator : Logic  Inputs=6  AllPortsSameDT=off  OutDataTypeStr=boolean
  FAULT_Logical Operator{,1..3} (4 alike) : F_Line_block/Subsystem
  FAULT_Logical Operator_{2..6} (5 alike) : F_Line_block/Subsystem
  Logical Operator1 : Logic  AllPortsSameDT=off  OutDataTypeStr=boolean
  FAULT_Logical Operator1_2 : F_Line_block/Subsystem
  Logical Operator2 : Logic  Operator=OR  AllPortsSameDT=off  OutDataTypeStr=boolean
  FAULT_Logical Operator2_2 : F_Line_block/Subsystem
  Logical Operator3 : Logic  Inputs=4  AllPortsSameDT=off  OutDataTypeStr=boolean
  FAULT_Logical Operator3_2 : F_Line_block/Subsystem
  FAULT_Logical Operator3_3 : F_Line_block/Subsystem
  FAULT_Logical Operator3_4 : F_Line_block/Subsystem
  Mux5 : Mux  Inputs=2
  FAULT_Mux5 : F_Line_block/Subsystem
  FAULT_Mux5_2 : F_Line_block/Subsystem
  Selectpitchroll : Selector  InputPortWidth=3  IndexOptions=Index vector (dialog)  Indices=[2 3]  OutputSizes=1
  FAULT_Selectpitchroll : F_Line_block/Subsystem
  maxdw1 : simulink/Logic and Bit Operations/Compare To Constant  relop=<=  const=Estimator.pos.ofDPQMax  OutDataTypeStr=boolean
  FAULT_maxdw1 : F_Line_block/Subsystem
  maxdw2 : simulink/Logic and Bit Operations/Compare To Constant  relop=<=  const=Estimator.pos.ofDPQMax  OutDataTypeStr=boolean
  FAULT_maxdw2 : F_Line_block/Subsystem
  maxp : simulink/Logic and Bit Operations/Compare To Constant  relop=<=  const=Estimator.pos.ofPitchRollMax  OutDataTypeStr=boolean
  FAULT_maxp : F_Line_block/Subsystem
  maxp2 : simulink/Logic and Bit Operations/Compare To Constant  relop=<=  const=Estimator.pos.ofPQHovMax  OutDataTypeStr=boolean
  FAULT_maxp2 : F_Line_block/Subsystem
  maxq : simulink/Logic and Bit Operations/Compare To Constant  relop=<=  const=Estimator.pos.ofPitchRollMax  OutDataTypeStr=boolean
  FAULT_maxq : F_Line_block/Subsystem
  maxq2 : simulink/Logic and Bit Operations/Compare To Constant  relop=<=  const=Estimator.pos.ofPQHovMax  OutDataTypeStr=boolean
  FAULT_maxq2 : F_Line_block/Subsystem
  maxw1 : simulink/Logic and Bit Operations/Compare To Constant  relop=<=  const=Estimator.pos.ofPQMax  OutDataTypeStr=boolean
  FAULT_maxw{1..4} (4 alike) : F_Line_block/Subsystem
  maxw2 : simulink/Logic and Bit Operations/Compare To Constant  relop=<=  const=Estimator.pos.ofPQMax  OutDataTypeStr=boolean
  maxw3 : simulink/Logic and Bit Operations/Compare To Constant  relop=<=  const=Estimator.pos.deltaDXYMax  OutDataTypeStr=boolean
  maxw4 : simulink/Logic and Bit Operations/Compare To Constant  relop=<=  const=Estimator.pos.deltaDXYMax  OutDataTypeStr=boolean
  minHeightforOF : simulink/Logic and Bit Operations/Compare To Constant  relop=<=  const=Estimator.pos.opticalFlowZMax  OutDataTypeStr=boolean
  FAULT_minHeightforOF : F_Line_block/Subsystem
  enable_flag : Outport
  FAULT_enable_flag : F_Line_block/Subsystem
  wires:
  minHeightforOF/1 -> FAULT_Logical Operator3_4/1
  FAULT_Logical Operator3_4/1 -> Logical Operator3/4
  IIRgyroz/1 -> FAULT_DiscreteDerivative/1
  FAULT_DiscreteDerivative/1 -> DiscreteDerivative/1
  Mux5/1 -> FAULT_Demux1/1, FAULT_IIRgyroz/1, Demux4/1
  maxw4/1 -> FAULT_Logical Operator3_3/1
  FAULT_Logical Operator3_3/1 -> Logical Operator3/3
  maxw3/1 -> FAULT_Logical Operator3_2/1
  FAULT_Logical Operator3_2/1 -> Logical Operator3/2
  dxyOF_datin/1 -> FAULT_Add/1
  FAULT_Add/1 -> Add/1
  Demux3/2 -> FAULT_Abs9/1
  FAULT_Abs9/1 -> Abs9/1
  Demux3/1 -> FAULT_Abs8/1
  FAULT_Abs8/1 -> Abs8/1
  dxy_estimin/1 -> FAULT_Add_2/1
  FAULT_Add_2/1 -> Add/2
  Add/1 -> FAULT_Demux3/1
  FAULT_Demux3/1 -> Demux3/1
  Abs9/1 -> FAULT_maxw4/1
  FAULT_maxw4/1 -> maxw4/1
  Abs8/1 -> FAULT_maxw3/1
  FAULT_maxw3/1 -> maxw3/1
  Logical Operator2/1 -> FAULT_Logical Operator3/1
  FAULT_Logical Operator3/1 -> Logical Operator3/1
  Logical Operator3/1 -> FAULT_enable_flag/1
  FAULT_enable_flag/1 -> enable_flag/1
  DiscreteDerivative/1 -> FAULT_Demux2/1  "dpq"
  FAULT_Demux2/1 -> Demux2/1
  Demux2/2 -> FAULT_Abs7/1
  FAULT_Abs7/1 -> Abs7/1
  Demux2/1 -> FAULT_Abs6/1
  FAULT_Abs6/1 -> Abs6/1
  Abs7/1 -> FAULT_maxdw2/1
  FAULT_maxdw2/1 -> maxdw2/1
  Abs6/1 -> FAULT_maxdw1/1
  FAULT_maxdw1/1 -> maxdw1/1
  Logical Operator1/1 -> FAULT_Logical Operator2_2/1
  FAULT_Logical Operator2_2/1 -> Logical Operator2/2
  Demux1/2 -> FAULT_Abs5/1
  FAULT_Abs5/1 -> Abs5/1
  Demux1/1 -> FAULT_Abs4/1
  FAULT_Abs4/1 -> Abs4/1
  Abs5/1 -> FAULT_maxq2/1
  FAULT_maxq2/1 -> maxq2/1
  Abs4/1 -> FAULT_maxp2/1
  FAULT_maxp2/1 -> maxp2/1
  Abs3/1 -> FAULT_maxq/1
  FAULT_maxq/1 -> maxq/1
  Abs2/1 -> FAULT_maxp/1
  FAULT_maxp/1 -> maxp/1
  Demux4/2 -> FAULT_Abs1/1
  FAULT_Abs1/1 -> Abs1/1
  Demux4/1 -> FAULT_Abs/1
  FAULT_Abs/1 -> Abs/1
  Abs1/1 -> FAULT_maxw2/1
  FAULT_maxw2/1 -> maxw2/1
  Abs/1 -> FAULT_maxw1/1
  FAULT_maxw1/1 -> maxw1/1
  Z_estimin/1 -> FAULT_minHeightforOF/1
  FAULT_minHeightforOF/1 -> minHeightforOF/1
  Logical Operator/1 -> FAULT_Logical Operator2/1
  FAULT_Logical Operator2/1 -> Logical Operator2/1
  maxw1/1 -> FAULT_Logical Operator_3/1
  FAULT_Logical Operator_3/1 -> Logical Operator/3
  Bus Selector/1 -> FAULT_Mux5/1  "<p>"
  FAULT_Mux5/1 -> Mux5/1
  Selectpitchroll/1 -> FAULT_Demux5/1
  FAULT_Demux5/1 -> Demux5/1
  sensorIMU_datin/1 -> Bus Selector/1
  maxq2/1 -> FAULT_Logical Operator1_2/1
  FAULT_Logical Operator1_2/1 -> Logical Operator1/2
  Bus Selector/2 -> FAULT_Mux5_2/1  "<q>"
  FAULT_Mux5_2/1 -> Mux5/2
  maxp/1 -> FAULT_Logical Operator/1
  FAULT_Logical Operator/1 -> Logical Operator/1
  maxw2/1 -> FAULT_Logical Operator_4/1
  FAULT_Logical Operator_4/1 -> Logical Operator/4
  orient_estimin/1 -> FAULT_Selectpitchroll/1
  FAULT_Selectpitchroll/1 -> Selectpitchroll/1
  maxdw1/1 -> FAULT_Logical Operator_5/1
  FAULT_Logical Operator_5/1 -> Logical Operator/5
  maxdw2/1 -> ?
  FAULT_Logical Operator_5/1 -> Logical Operator/5
  maxq/1 -> FAULT_Logical Operator_2/1
  FAULT_Logical Operator_2/1 -> Logical Operator/2
  Demux5/1 -> FAULT_Abs2/1
  FAULT_Abs2/1 -> Abs2/1
  Demux5/2 -> FAULT_Abs3/1
  FAULT_Abs3/1 -> Abs3/1
  maxp2/1 -> FAULT_Logical Operator1/1
  FAULT_Logical Operator1/1 -> Logical Operator1/1

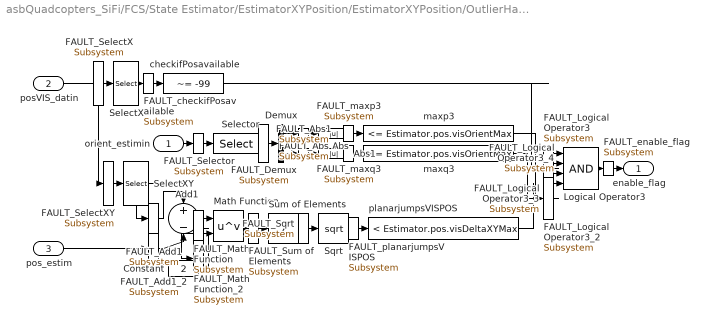
== system asbQuadcopters_SiFi/FCS/State Estimator/EstimatorXYPosition/EstimatorXYPosition/OutlierHandling ==
  orient_estimin : Inport
  posVIS_datin : Inport  Port=2
  pos_estim : Inport  Port=3
  Abs : Abs
  FAULT_Abs : F_Line_block/Subsystem
  Abs1 : Abs
  FAULT_Abs1 : F_Line_block/Subsystem
  Add1 : Sum  Inputs=+-  AccumDataTypeStr=single
  FAULT_Add1 : F_Line_block/Subsystem
  FAULT_Add1_2 : F_Line_block/Subsystem
  Constant : Constant  Value=2  OutDataTypeStr=single
  Demux : Demux  Outputs=2
  FAULT_Demux : F_Line_block/Subsystem
  Logical Operator3 : Logic  Inputs=4  AllPortsSameDT=off  OutDataTypeStr=boolean
  FAULT_Logical Operator3 : F_Line_block/Subsystem
  FAULT_Logical Operator3_2 : F_Line_block/Subsystem
  FAULT_Logical Operator3_3 : F_Line_block/Subsystem
  FAULT_Logical Operator3_4 : F_Line_block/Subsystem
  Math Function : Math  Operator=pow  SaturateOnIntegerOverflow=on
  FAULT_Math Function : F_Line_block/Subsystem
  FAULT_Math Function_2 : F_Line_block/Subsystem
  SelectX : Selector  InputPortWidth=4  IndexOptions=Index vector (dialog)  Indices=[1]  OutputSizes=1
  FAULT_SelectX : F_Line_block/Subsystem
  SelectXY : Selector  InputPortWidth=4  IndexOptions=Index vector (dialog)  Indices=[1 2]  OutputSizes=1
  FAULT_SelectXY : F_Line_block/Subsystem
  Selector : Selector  InputPortWidth=3  IndexOptions=Index vector (dialog)  Indices=[2 3]  OutputSizes=1
  FAULT_Selector : F_Line_block/Subsystem
  Sqrt : Sqrt  SaturateOnIntegerOverflow=on
  FAULT_Sqrt : F_Line_block/Subsystem
  Sum of Elements : Sum  Inputs=+
  FAULT_Sum of Elements : F_Line_block/Subsystem
  checkifPosavailable : simulink/Logic and Bit Operations/Compare To Constant  relop=~=  const=-99  OutDataTypeStr=boolean
  FAULT_checkifPosavailable : F_Line_block/Subsystem
  maxp3 : simulink/Logic and Bit Operations/Compare To Constant  relop=<=  const=Estimator.pos.visOrientMax  OutDataTypeStr=boolean
  FAULT_maxp3 : F_Line_block/Subsystem
  maxq3 : simulink/Logic and Bit Operations/Compare To Constant  relop=<=  const=Estimator.pos.visOrientMax  OutDataTypeStr=boolean
  FAULT_maxq3 : F_Line_block/Subsystem
  planarjumpsVISPOS : simulink/Logic and Bit Operations/Compare To Constant  relop=<  const=Estimator.pos.visDeltaXYMax  OutDataTypeStr=boolean
  FAULT_planarjumpsVISPOS : F_Line_block/Subsystem
  enable_flag : Outport
  FAULT_enable_flag : F_Line_block/Subsystem
  wires:
  Abs1/1 -> FAULT_maxq3/1
  FAULT_maxq3/1 -> maxq3/1
  Abs/1 -> FAULT_maxp3/1
  FAULT_maxp3/1 -> maxp3/1
  Demux/2 -> FAULT_Abs1/1
  FAULT_Abs1/1 -> Abs1/1
  Demux/1 -> FAULT_Abs/1
  FAULT_Abs/1 -> Abs/1
  Selector/1 -> FAULT_Demux/1
  FAULT_Demux/1 -> Demux/1
  orient_estimin/1 -> FAULT_Selector/1
  FAULT_Selector/1 -> Selector/1
  planarjumpsVISPOS/1 -> FAULT_Logical Operator3_4/1
  FAULT_Logical Operator3_4/1 -> Logical Operator3/4
  Sqrt/1 -> FAULT_planarjumpsVISPOS/1
  FAULT_planarjumpsVISPOS/1 -> planarjumpsVISPOS/1
  pos_estim/1 -> FAULT_Add1_2/1
  FAULT_Add1_2/1 -> Add1/2
  Add1/1 -> FAULT_Math Function/1
  FAULT_Math Function/1 -> Math Function/1
  SelectXY/1 -> FAULT_Add1/1
  FAULT_Add1/1 -> Add1/1
  maxq3/1 -> FAULT_Logical Operator3_3/1
  FAULT_Logical Operator3_3/1 -> Logical Operator3/3
  maxp3/1 -> FAULT_Logical Operator3_2/1
  FAULT_Logical Operator3_2/1 -> Logical Operator3/2
  Logical Operator3/1 -> FAULT_enable_flag/1
  FAULT_enable_flag/1 -> enable_flag/1
  checkifPosavailable/1 -> FAULT_Logical Operator3/1
  FAULT_Logical Operator3/1 -> Logical Operator3/1
  SelectX/1 -> FAULT_checkifPosavailable/1
  FAULT_checkifPosavailable/1 -> checkifPosavailable/1
  posVIS_datin/1 -> FAULT_SelectX/1, FAULT_SelectXY/1
  FAULT_SelectX/1 -> SelectX/1
  FAULT_SelectXY/1 -> SelectXY/1
  Sum of Elements/1 -> FAULT_Sqrt/1
  FAULT_Sqrt/1 -> Sqrt/1
  Constant/1 -> FAULT_Math Function_2/1
  FAULT_Math Function_2/1 -> Math Function/2
  Math Function/1 -> FAULT_Sum of Elements/1
  FAULT_Sum of Elements/1 -> Sum of Elements/1

== system asbQuadcopters_SiFi/Sensor/Sensor System/IMU_Pressure/HAL_acquisition_creator/HAL_acc_SI_creator ==
  x : Inport
  y : Inport  Port=2
  z : Inport  Port=3
  Bus Creator : BusCreator  Inputs=4  OutDataTypeStr=Bus: HAL_acc_SI_t
  temperature : Constant  Value=0  OutDataTypeStr=single
  HAL_acc_SI : Outport
  wires:
  temperature/1 -> Bus Creator/4  "temperature"
  Bus Creator/1 -> HAL_acc_SI/1  "HAL_acc_SI"
  x/1 -> Bus Creator/1
  y/1 -> Bus Creator/2
  z/1 -> Bus Creator/3

== system asbQuadcopters_SiFi/Sensor/Sensor System/IMU_Pressure/HAL_acquisition_creator/HAL_fifo_gyro_SI_t_creator ==
  Bus Creator : BusCreator  Inputs=3  OutDataTypeStr=Bus: HAL_fifo_gyro_SI_t  NonVirtualBus=on
      settings: InheritFromInputs=off
  Vector Concatenate : Concatenate  NumInputs=5
  z : Constant  Value=0  OutDataTypeStr=single
  z1 : Constant  Value=0  OutDataTypeStr=single
  z2 : Constant  Value=0  OutDataTypeStr=single
  HAL_fifo_gyro_SI_TempCorr : Outport  PortDimensions=5  LockScale=on
  wires:
  z1/1 -> Bus Creator/2  "y"
  Bus Creator/1 -> Vector Concatenate/3, Vector Concatenate/4, Vector Concatenate/5, Vector Concatenate/2, Vector Concatenate/1  "HAL_fifo_gyro_SI_TempCorr"
  Vector Concatenate/1 -> HAL_fifo_gyro_SI_TempCorr/1
  z/1 -> Bus Creator/3  "z"
  z2/1 -> Bus Creator/1  "x"

== system asbQuadcopters_SiFi/Sensor/Sensor System/IMU_Pressure/HAL_acquisition_creator/HAL_fifo_gyro_SI_t_creator1 ==
  Bus Creator : BusCreator  Inputs=3  OutDataTypeStr=Bus: HAL_fifo_gyro_SI_t  NonVirtualBus=on
      settings: InheritFromInputs=off
  Vector Concatenate : Concatenate  NumInputs=5
  x : Constant  Value=0  OutDataTypeStr=single
  x1 : Constant  Value=0  OutDataTypeStr=single
  x2 : Constant  Value=0  OutDataTypeStr=single
  HAL_fifo_acce_SI_TempCorr : Outport  PortDimensions=5  LockScale=on
  wires:
  x1/1 -> Bus Creator/2  "y"
  Bus Creator/1 -> Vector Concatenate/5, Vector Concatenate/4, Vector Concatenate/3, Vector Concatenate/2, Vector Concatenate/1  "HAL_fifo_gyro_SI_TempCorr"
  x2/1 -> Bus Creator/3  "z"
  x/1 -> Bus Creator/1  "x"
  Vector Concatenate/1 -> HAL_fifo_acce_SI_TempCorr/1

== system asbQuadcopters_SiFi/Sensor/Sensor System/IMU_Pressure/HAL_acquisition_creator/HAL_fifo_gyro_SI_t_creator2 ==
  Bus Creator : BusCreator  Inputs=3  OutDataTypeStr=Bus: HAL_fifo_gyro_SI_t  NonVirtualBus=on
      settings: InheritFromInputs=off
  Vector Concatenate : Concatenate  NumInputs=5
  z : Constant  Value=0  OutDataTypeStr=single
  z1 : Constant  Value=0  OutDataTypeStr=single
  z2 : Constant  Value=0  OutDataTypeStr=single
  HAL_fifo_gyro_SI_TempCorr : Outport  PortDimensions=5  LockScale=on
  wires:
  Vector Concatenate/1 -> HAL_fifo_gyro_SI_TempCorr/1
  Bus Creator/1 -> Vector Concatenate/3, Vector Concatenate/4, Vector Concatenate/5, Vector Concatenate/2, Vector Concatenate/1  "HAL_fifo_gyro_SI_TempCorr"
  z/1 -> Bus Creator/3  "z"
  z2/1 -> Bus Creator/1  "x"
  z1/1 -> Bus Creator/2  "y"
